simulink model "rotpentemplate"  (R2021b)
settings: Solver=VariableStepDiscrete  StartTime=0.0  StopTime=120  RelTol=1e-3  EnableMultiTasking=on
undefined symbols (not defined in the file or in its folder): adingain, adinoffs, daoutgain, daoutoffs, DiscIntNeverNeededParam, Discrete, h, K_lqr, sys_dis, Time
libraries: simulink x5, ctrlSharedLib x2
settings Model: Creator=rbabuska  LastModifiedBy=ellyb
settings SolverCC: AlgebraicLoopSolver=TrustRegion
settings DataIOCC: LimitDataPoints=on  SaveFormat=Array  ReturnWorkspaceOutputs=off  SignalLoggingName=sigsOut
settings OptimizationCC: BooleanDataType=off  ExpressionDepthLimit=2147483647  InitFltsAndDblsToZero=on  LifeSpan=inf
settings DebuggingCC: SaveWithParameterizedLinksMsg=none  SignalResolutionControl=TryResolveAllWithWarning  MultiTaskDSMMsg=warning  MultiTaskCondExecSysMsg=none  AllowSymbolicDim=off  StateNameClashWarn=warning  SFUnexpectedBacktrackingDiag=warning  SFNoUnconditionalDefaultTransitionDiag=warning  SFExecutionAtInitializationDiag=none  ArithmeticOperatorsInVariantConditions=warning
settings HardwareCC: ProdBitPerPointer=32  ProdBitPerSizeT=32  ProdBitPerPtrDiffT=32  ProdLargestAtomicFloat=None  ProdIntDivRoundTo=Undefined  ProdEndianess=Unspecified  ProdWordSize=32  ProdHWDeviceType=32-bit Generic  TargetUnknown=on
settings ModelReferenceCC: PropagateSignalLabelsOutOfModel=off
settings SFSimCC: SimUseLocalCustomCode=off  CustomCodeUndefinedFunction=UseInterfaceOnly
settings RTWCC: RTWUseLocalCustomCode=off
settings CodeAppCC: StateflowObjectComments=on
settings GRTTargetCC: TargetFcnLib=ansi_tfl_tmw.mat  TargetLangStandard=C89/C90 (ANSI)  CombineOutputUpdateFcns=off  GRTInterface=on
settings ConfigComp: CovMetricSettings=dw  CovSaveCumulativeToWorkspaceVar=on  CovSaveSingleToWorkspaceVar=on  CovExternalEMLEnable=off

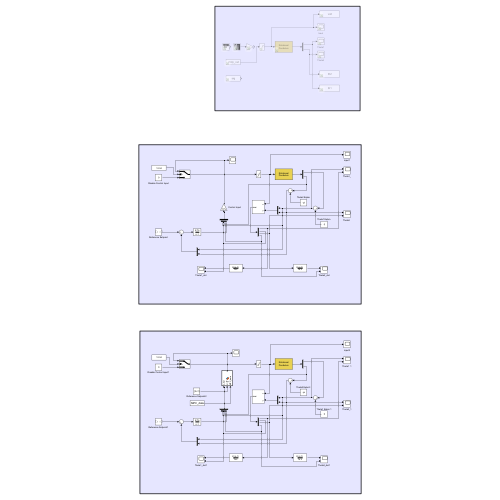
[thumbnail: Simulink's stored preview of the top-level diagram]
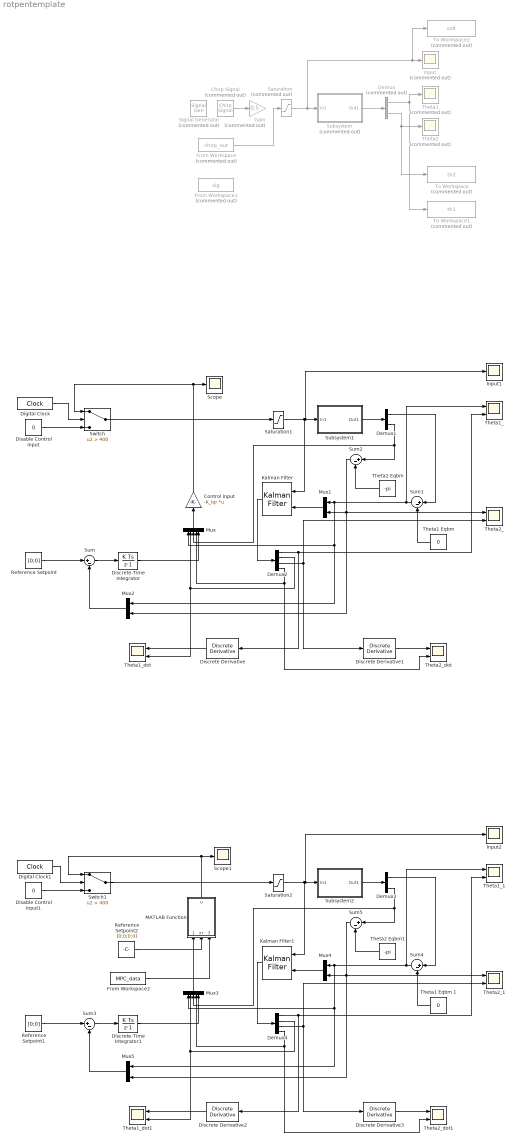
== system rotpentemplate ==
  Chirp Signal : simulink/Sources/Chirp Signal  Commented=on  f1=2  T=45  f2=6
  Control Input : Gain  Gain=-K_lqr  Multiplication=Matrix(K*u)
  Demux : Demux  Commented=on  Outputs=2
  Demux1 : Demux  Outputs=2
  Demux2 : Demux
  Demux3 : Demux  Outputs=2
  Demux4 : Demux
  Digital Clock : DigitalClock  SampleTime=h
  Digital Clock1 : DigitalClock  SampleTime=h
  Disable Control Input : Constant  Value=0  SampleTime=-1
  Disable Control Input1 : Constant  Value=0  SampleTime=-1
  Discrete Derivative{,1..3} (4 alike) : simulink/Discrete/Discrete Derivative  gainval=1.0  ICPrevScaledInput=0.0  OutMin=[]  OutMax=[]  OutDataType=fixdt(1, 16)  OutScaling=2^-10  DoSatur=off
  Discrete-Time Integrator : DiscreteIntegrator  SampleTime=h  ICPrevOutput=DiscIntNeverNeededParam  ICPrevScaledInput=DiscIntNeverNeededParam
  Discrete-Time Integrator1 : DiscreteIntegrator  SampleTime=h  ICPrevOutput=DiscIntNeverNeededParam  ICPrevScaledInput=DiscIntNeverNeededParam
  From Workspace : FromWorkspace  Commented=on  VariableName=chirp_out  SampleTime=h
  From Workspace1 : FromWorkspace  Commented=on  VariableName=sig  SampleTime=h
  From Workspace2 : FromWorkspace  VariableName=MPC_data  SampleTime=h
  Gain : Gain  Commented=on  Gain=0.5
  Input : Scope  Commented=on
  Input1 : Scope
  Input2 : Scope
  Kalman Filter : ctrlSharedLib/Kalman Filter  TimeDomain=Discrete-Time  UseCurrentEstimator=on  ModelSource=Individual A, B, C, D matrices  ModelSourceVariable=ss(0.95,1,1,0,1)  A=sys_dis.A  B=sys_dis.B  C=sys_dis.C  D=sys_dis.D  NumberOfStates=1  NumberOfInputs=1  NumberOfOutputs=1  InitialEstimateSource=Dialog  X0=0  P0=10  UseK=off  UseGH=off  NumberOfProcessNoiseInputs=1  G=1  TimeInvariantG=on  H=0  TimeInvariantH=on  Q=diag([0.1^2 0.1^2 0.01^2 0.001^2])  TimeInvariantQ=on  R=diag([0.01^2 0.05^2])  TimeInvariantR=on  N=0  TimeInvariantN=on  AddInputPort=on  AddEnablePort=off  OutputEstimatedY=off  OutputP=off  Ts=-1
  Kalman Filter1 : ctrlSharedLib/Kalman Filter  TimeDomain=Discrete-Time  UseCurrentEstimator=on  ModelSource=Individual A, B, C, D matrices  ModelSourceVariable=ss(0.95,1,1,0,1)  A=sys_dis.A  B=sys_dis.B  C=sys_dis.C  D=sys_dis.D  NumberOfStates=1  NumberOfInputs=1  NumberOfOutputs=1  InitialEstimateSource=Dialog  X0=0  P0=10  UseK=off  UseGH=off  NumberOfProcessNoiseInputs=1  G=1  TimeInvariantG=on  H=0  TimeInvariantH=on  Q=diag([0.1^2 0.1^2 0.01^2 0.001^2])  TimeInvariantQ=on  R=diag([0.01^2 0.05^2])  TimeInvariantR=on  N=0  TimeInvariantN=on  AddInputPort=on  AddEnablePort=off  OutputEstimatedY=off  OutputP=off  Ts=-1
  MATLAB Function : MATLAB Function  TreatAsAtomicUnit=on
  Mux : Mux  Inputs=5
  Mux{1..2,4..5} (4 alike) : Mux  Inputs=2
  Mux3 : Mux  Inputs=5
  Reference Setpoint : Constant  Value=[0;0]  SampleTime=-1
  Reference Setpoint1 : Constant  Value=[0;0]  SampleTime=-1
  Reference Setpoint2 : Constant  Value=[0;0;0;0]  SampleTime=-1
  Saturation : Saturate  Commented=on  UpperLimit=1  LowerLimit=-1
  Saturation1 : Saturate  UpperLimit=1  LowerLimit=-1
  Saturation2 : Saturate  UpperLimit=1  LowerLimit=-1
  Scope : Scope
  Scope1 : Scope
  Signal Generator : SignalGenerator  Commented=on  Amplitude=0.3*1
  Subsystem : Subsystem  Commented=on
      mask Display: disp('Rotational\nPendulum')
  Subsystem1 : Subsystem
      mask Display: disp('Rotational\nPendulum')
  Subsystem2 : Subsystem
      mask Display: disp('Rotational\nPendulum')
  Sum{,1..5} (6 alike) : Sum  Inputs=|+-
  Switch : Switch  Criteria=u2 > Threshold  Threshold=400
  Switch1 : Switch  Criteria=u2 > Threshold  Threshold=400
  Theta1 : Scope  Commented=on
  "Theta1 Eqbm " : Constant  Value=0  SampleTime=-1
  Theta1 Eqbm 1 : Constant  Value=0  SampleTime=-1
  Theta1_ : Scope  NumInputPorts=2
  Theta1_1 : Scope  NumInputPorts=2
  Theta1_dot : Scope  NumInputPorts=2
  Theta1_dot1 : Scope  NumInputPorts=2
  Theta2 : Scope  Commented=on
  Theta2 Eqbm : Constant  Value=-pi  SampleTime=-1
  Theta2 Eqbm1 : Constant  Value=-pi  SampleTime=-1
  Theta2_ : Scope  NumInputPorts=2
  Theta2_1 : Scope  NumInputPorts=2
  Theta2_dot : Scope  NumInputPorts=2
  Theta2_dot1 : Scope  NumInputPorts=2
  To Workspace : ToWorkspace  Commented=on  VariableName=th2  SaveFormat=Timeseries  SampleTime=-1
  To Workspace1 : ToWorkspace  Commented=on  VariableName=th1  SaveFormat=Timeseries  SampleTime=-1
  To Workspace2 : ToWorkspace  Commented=on  VariableName=volt  SaveFormat=Timeseries  SampleTime=-1
  wires:
  Saturation/1 -> Subsystem/1(In1), To Workspace2/1, Input/1
  Subsystem/1(Out1) -> Demux/1
  Demux/1 -> To Workspace1/1, Theta1/1
  Demux/2 -> To Workspace/1, Theta2/1
  Chirp Signal/1 -> Gain/1
  From Workspace/1 -> Saturation/1
  Demux1/1 -> Sum1/1
  Demux1/2 -> Sum2/1, Mux/3
  Subsystem1/1(Out1) -> Demux1/1
  Saturation1/1 -> Subsystem1/1(In1), Input1/1, Kalman Filter/1
  Kalman Filter/1 -> Demux2/1
  Demux2/3 -> Theta2_/2, Discrete Derivative1/1
  Mux/1 -> Control Input/1
  Demux2/2 -> Theta1_dot/2, Mux/2
  Demux2/1 -> Theta1_/2, Discrete Derivative/1
  Demux2/4 -> Theta2_dot/2, Mux/4
  "Theta1 Eqbm "/1 -> Sum1/2
  Mux1/1 -> Kalman Filter/2
  Discrete Derivative1/1 -> Theta2_dot/1
  Discrete Derivative/1 -> Theta1_dot/1
  Theta2 Eqbm/1 -> Sum2/2
  Sum2/1 -> Mux1/2, Mux2/2, Theta2_/1
  Sum1/1 -> Mux2/1, Mux/1, Mux1/1, Theta1_/1
  Switch/1 -> Saturation1/1
  Control Input/1 -> Scope/1, Switch/1
  Digital Clock/1 -> Switch/2
  Disable Control Input/1 -> Switch/3
  Sum/1 -> Discrete-Time Integrator/1
  Mux2/1 -> Sum/2
  Reference Setpoint/1 -> Sum/1
  Discrete-Time Integrator/1 -> Mux/5
  Discrete-Time Integrator1/1 -> Mux3/5
  Sum3/1 -> Discrete-Time Integrator1/1
  Reference Setpoint1/1 -> Sum3/1
  Mux5/1 -> Sum3/2
  Demux4/4 -> Theta2_dot1/2, Mux3/4
  Saturation2/1 -> Subsystem2/1(In1), Input2/1, Kalman Filter1/1
  Sum5/1 -> Mux4/2, Mux5/2, Theta2_1/1
  Sum4/1 -> Mux5/1, Mux3/1, Mux4/1, Theta1_1/1
  Demux4/2 -> Theta1_dot1/2, Mux3/2
  Theta2 Eqbm1/1 -> Sum5/2
  Discrete Derivative2/1 -> Theta1_dot1/1
  Switch1/1 -> Saturation2/1
  Theta1 Eqbm 1/1 -> Sum4/2
  MATLAB Function/1(u) -> Switch1/1, Scope1/1
  Subsystem2/1(Out1) -> Demux3/1
  Disable Control Input1/1 -> Switch1/3
  Kalman Filter1/1 -> Demux4/1
  Digital Clock1/1 -> Switch1/2
  Discrete Derivative3/1 -> Theta2_dot1/1
  Mux4/1 -> Kalman Filter1/2
  Mux3/1 -> MATLAB Function/1(x_hat)
  Demux4/1 -> Theta1_1/2, Discrete Derivative2/1
  Demux3/1 -> Sum4/1
  Demux3/2 -> Sum5/1, Mux3/3
  Demux4/3 -> Theta2_1/2, Discrete Derivative3/1
  From Workspace2/1 -> MATLAB Function/3(MPC_data)
  Reference Setpoint2/1 -> MATLAB Function/2(xr)

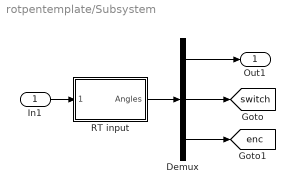
== system rotpentemplate/Subsystem ==
  In1 : Inport
  Demux : Demux  Outputs=[2 4 1]
  RT input : Subsystem  mask{Ts=h, channels=[6 7]}
      mask prompts: Ts "Sample time [s]:"; channels "Channels to read (e.g., [6 7])"
      mask init:
      | hwinit;
      | 
      | % initialize FPGA
      | fugihandle = fugiboard('Open', 'Pendulum1');
      | fugihandle.WatchdogTimeout = 0.5;
      | fugiboard('SetParams', fugihandle);
      | fugiboard('Write', fugihandle, 0, 0, 0, 0);  % dummy write to sync interface board
      | fugiboard('Write', fugihandle, 5, 1, 0, 0);  % reset position, activate relay
      | data = fugiboard('Read', fugihandle);        % get version info from FPGA
      | % model = bitshift(data(1), -5); 
      | % version = bitand(data(1), 31);
      | % disp(sprintf('FPGA setup %d, version %d', model, version)); % for the B&P it should say 1 1, or else there is a problem
      | fugiboard('Write', fugihandle, 0, 1, 0, 0);  % end reset
      | pause(0.1);                         % give relay some time to respond
      mask Display: disp('Rotational\nPendulum')
  Out1 : Outport
  tag scope: enc=global, switch=global
  wires:
  RT input/1(Angles) -> Demux/1
  Demux/1 -> Out1/1
  Demux/2 -> [switch]
  Demux/3 -> [enc]
  In1/1 -> RT input/1(Motors)

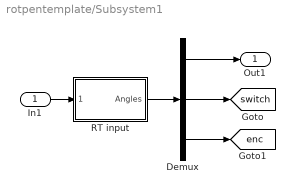
== system rotpentemplate/Subsystem1 ==
  In1 : Inport
  Demux : Demux  Outputs=[2 4 1]
  RT input : Subsystem  mask{Ts=h, channels=[6 7]}
      mask prompts: Ts "Sample time [s]:"; channels "Channels to read (e.g., [6 7])"
      mask init: same as rotpentemplate/Subsystem/RT input
      mask Display: disp('Rotational\nPendulum')
  Out1 : Outport
  tag scope: enc=global, switch=global
  wires:
  RT input/1(Angles) -> Demux/1
  Demux/1 -> Out1/1
  Demux/2 -> [switch]
  Demux/3 -> [enc]
  In1/1 -> RT input/1(Motors)

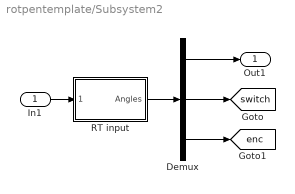
== system rotpentemplate/Subsystem2 ==
  In1 : Inport
  Demux : Demux  Outputs=[2 4 1]
  RT input : Subsystem  mask{Ts=h, channels=[6 7]}
      mask prompts: Ts "Sample time [s]:"; channels "Channels to read (e.g., [6 7])"
      mask init: same as rotpentemplate/Subsystem/RT input
      mask Display: disp('Rotational\nPendulum')
  Out1 : Outport
  tag scope: enc=global, switch=global
  wires:
  RT input/1(Angles) -> Demux/1
  Demux/1 -> Out1/1
  Demux/2 -> [switch]
  Demux/3 -> [enc]
  In1/1 -> RT input/1(Motors)

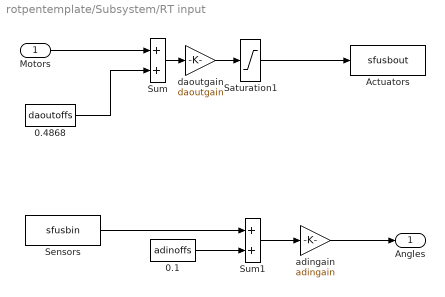
== system rotpentemplate/Subsystem/RT input ==
  Motors : Inport
  0.1 : Constant  Value=adinoffs
  0.4868 : Constant  Value=daoutoffs
  Actuators : S-Function  FunctionName=sfusbout  Parameters=Ts, fugihandle  SFunctionDeploymentMode=off  EnableBusSupport=off
  Saturation1 : Saturate  UpperLimit=10  LowerLimit=-10
  Sensors : S-Function  FunctionName=sfusbin  Parameters=Ts, fugihandle, channels  SFunctionDeploymentMode=off  EnableBusSupport=off
  Sum : Sum  InputSameDT=on  SaturateOnIntegerOverflow=on  OutDataTypeStr=Inherit: Same as first input
  Sum1 : Sum  InputSameDT=on  SaturateOnIntegerOverflow=on  OutDataTypeStr=Inherit: Same as first input
  adingain : Gain  Gain=adingain  SaturateOnIntegerOverflow=on  OutDataTypeStr=Inherit: Same as input  ParamDataTypeStr=Inherit: Same as input
  daoutgain : Gain  Gain=daoutgain  SaturateOnIntegerOverflow=on  OutDataTypeStr=Inherit: Same as input  ParamDataTypeStr=Inherit: Same as input
  Angles : Outport
  wires:
  Sum/1 -> daoutgain/1
  0.4868/1 -> Sum/2
  Motors/1 -> Sum/1
  Sum1/1 -> adingain/1
  0.1/1 -> Sum1/2
  adingain/1 -> Angles/1
  Saturation1/1 -> Actuators/1
  daoutgain/1 -> Saturation1/1
  Sensors/1 -> Sum1/1

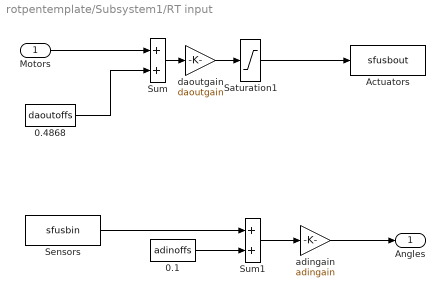
== system rotpentemplate/Subsystem1/RT input ==
  Motors : Inport
  0.1 : Constant  Value=adinoffs
  0.4868 : Constant  Value=daoutoffs
  Actuators : S-Function  FunctionName=sfusbout  Parameters=Ts, fugihandle  SFunctionDeploymentMode=off  EnableBusSupport=off
  Saturation1 : Saturate  UpperLimit=10  LowerLimit=-10
  Sensors : S-Function  FunctionName=sfusbin  Parameters=Ts, fugihandle, channels  SFunctionDeploymentMode=off  EnableBusSupport=off
  Sum : Sum  InputSameDT=on  SaturateOnIntegerOverflow=on  OutDataTypeStr=Inherit: Same as first input
  Sum1 : Sum  InputSameDT=on  SaturateOnIntegerOverflow=on  OutDataTypeStr=Inherit: Same as first input
  adingain : Gain  Gain=adingain  SaturateOnIntegerOverflow=on  OutDataTypeStr=Inherit: Same as input  ParamDataTypeStr=Inherit: Same as input
  daoutgain : Gain  Gain=daoutgain  SaturateOnIntegerOverflow=on  OutDataTypeStr=Inherit: Same as input  ParamDataTypeStr=Inherit: Same as input
  Angles : Outport
  wires:
  Sum/1 -> daoutgain/1
  0.4868/1 -> Sum/2
  Motors/1 -> Sum/1
  Sum1/1 -> adingain/1
  0.1/1 -> Sum1/2
  adingain/1 -> Angles/1
  Saturation1/1 -> Actuators/1
  daoutgain/1 -> Saturation1/1
  Sensors/1 -> Sum1/1

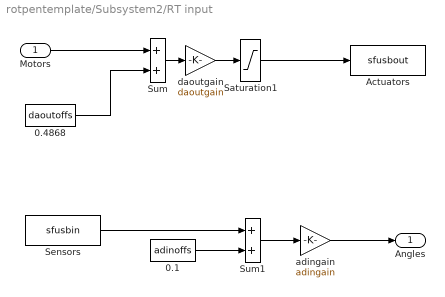
== system rotpentemplate/Subsystem2/RT input ==
  Motors : Inport
  0.1 : Constant  Value=adinoffs
  0.4868 : Constant  Value=daoutoffs
  Actuators : S-Function  FunctionName=sfusbout  Parameters=Ts, fugihandle  SFunctionDeploymentMode=off  EnableBusSupport=off
  Saturation1 : Saturate  UpperLimit=10  LowerLimit=-10
  Sensors : S-Function  FunctionName=sfusbin  Parameters=Ts, fugihandle, channels  SFunctionDeploymentMode=off  EnableBusSupport=off
  Sum : Sum  InputSameDT=on  SaturateOnIntegerOverflow=on  OutDataTypeStr=Inherit: Same as first input
  Sum1 : Sum  InputSameDT=on  SaturateOnIntegerOverflow=on  OutDataTypeStr=Inherit: Same as first input
  adingain : Gain  Gain=adingain  SaturateOnIntegerOverflow=on  OutDataTypeStr=Inherit: Same as input  ParamDataTypeStr=Inherit: Same as input
  daoutgain : Gain  Gain=daoutgain  SaturateOnIntegerOverflow=on  OutDataTypeStr=Inherit: Same as input  ParamDataTypeStr=Inherit: Same as input
  Angles : Outport
  wires:
  Sum/1 -> daoutgain/1
  0.4868/1 -> Sum/2
  Motors/1 -> Sum/1
  Sum1/1 -> adingain/1
  0.1/1 -> Sum1/2
  adingain/1 -> Angles/1
  Saturation1/1 -> Actuators/1
  daoutgain/1 -> Saturation1/1
  Sensors/1 -> Sum1/1

== matlab function rotpentemplate/MATLAB Function ==
  data: x_hat input; xr input; u output; MPC_data input
function u = fcn(x_hat, xr, MPC_data)

    % model_mpc = struct('A', A, 'B', B, 'C', C, 'Bd', zeros(size(B)), 'Cd', zeros(size(C, 1), 1), 'N', N);
    % constraint = Z.lqr;
    % penalty = struct('Q', Q, 'R', R, 'P', P);
    % terminal = Xn.lqr{1}; % LQR terminal set
    % mpcmats = []; % Calculated first time and then reused

    model_mpc = MPC_data.model;
    constraint = MPC_data.constraint;
    penalty = MPC_data.penalty;
    terminal = MPC_data.terminal; % LQR terminal set
    mpcmats = MPC_data.mpcmats; % Calculated first time and then reused


    % x0 = [0.25, 0, -0.1, 0]';  % initial condition for XN
    % %x0 = [0.2654; -3.0552; -0.1543; 5.2605];
    % xr = [0; 0; 0; 0]; % reference x_r set to 0 for regulation
    
    ref = [repmat([xr;0],N,1); xr];
    
    % x = zeros(dim.nx, size(T, 2));
    % x(:,1) = x0;
    model_mpc.x0 = x_hat(1:4);

    % usim = zeros(dim.nu, size(T, 2)-1);
    % V_N = zeros(size(T, 2)-1,1);
    % V_f = zeros(size(T, 2)-1,1);
    % l_xu = zeros(size(T, 2)-1,1);
    % l_xu0 = zeros(size(T, 2)-1,1);
    
    % t = zeros(size(T, 2)-1,1);
    
    
    % disp("MPC Regulation Started");
    % for k = 1:1:size(T, 2)-1
        % t(k) = (k-1) * h;
        % if ( k > 1 && (floor(t(k)) - floor(t(k-1))) == 1 )
        %     fprintf('t = %d sec \n', floor(t(k)));
        % end
    
        % Get the initial state from the non-linear dynamics last step state
        % model_mpc.x0 = x(:,k);
        [~, uk, ~, status, mpcmats] = linearmpc(xr,ref,0,model_mpc, constraint, penalty, ...
                                                 terminal, mpcmats);
        if status ~= 1
            disp("Error");
            % break;
        end
    
        % Get the first optimal control input from the MPC controller
        % usim(:,k) = uk(:,1);
        u = uk(:,1);
    
        % % Optimal cost function value
        % V_N(k) = FVAL;
    
        % if sm_nl_sys == 1
        %     % Simlulate the non-linear dynamics with the current control input for
        %     % Ts time (ZOH operation)
        %     tspan = [T(k), T(k+1)];
        %     x(:,k+1) = NLSystemDynamics(model, x_eq, x(:,k), tspan, usim(:, k));
        % else
        %     % Simlulate the linearized system
        %     x(:,k+1) = A*x(:,k) + B*usim(:,k);
        % end
    
        % Control Lyapunov function
        V_f(k) = 0.5*xk(:,end)'*P*xk(:,end);
    
        % Stage costs computed at different time steps
        l_xu(k) = 0.5*xk(:,end-1)'*Q*xk(:,end-1) + 0.5*uk(:,end)'*R*uk(:,end);
        l_xu0(k) = 0.5*xk(:,1)'*Q*xk(:,1) + 0.5*uk(:,1)'*R*uk(:,1);
    end
    
    
    
    
    y = u;
